simulink library "riscaldamento"  (R2024b)
settings: Solver=VariableStepAuto  StartTime=0.0  StopTime=10.0  RelTol=1e-3
settings Model: Creator=mainuser  LastModifiedBy=mainuser

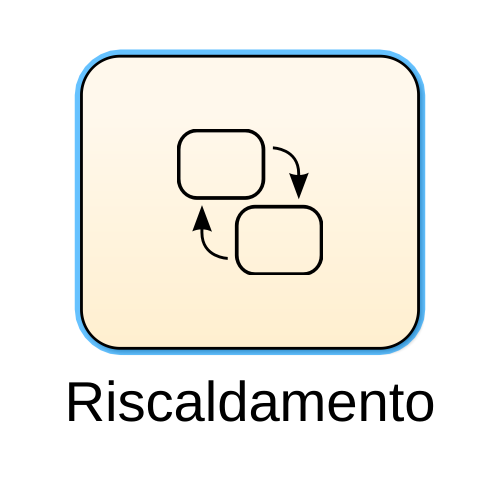
[thumbnail: Simulink's stored preview of the top-level diagram]
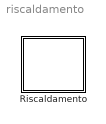
== system riscaldamento ==
  Riscaldamento : Stateflow chart  TreatAsAtomicUnit=on

== stateflow chart riscaldamento/Riscaldamento ==
